simulink model "SIM"  (R2020b)
settings: Solver=ode1  StartTime=0.0  StopTime=inf  FixedStep=0.005  RelTol=1e-3
values from neighbouring files (symbols this model uses):
  previous_input_to_hidden_layer = rand (K,1)* 0.2 - 0.1    [preparation.m]
  TableSIN = [0 0.0549778488291 0.109955562006 0.164933003878 0.219910038795 0.274886531105 0.32986234516 0.384837345313 0.439811395917 0.494784361331 0.549756105914 0.604726494028 ... (5001 elements, 5001x1)]    [TableSIN.mat]
  weights_Qj_model = rand (S,K)* 0.2 - 0.1    [preparation.m]
  weights_W2 = rand ( K+1 , R ) * 0.2 - 0.1    [preparation.m]
  weights_W3 = rand ( R+1 , W ) * 0.2 - 0.1    [preparation.m]
  weights_Wd_model = rand (K,1)* 0.2 - 0.1    [preparation.m]
  weights_Y1_model = rand (K,1)* 0.2 - 0.1    [preparation.m]
  weigths_W1 = rand ( S+1 , K ) * 0.2 - 0.1    [preparation.m]
undefined symbols (not defined in the file or in its folder): D, I, N, P, scaling_a, scaling_b, SkalB, SkalG, strengthening_PID, weights_W1_Model, weights_W2_Model, weights_Xj, WzmocnienieDoWyjscia
libraries: bur_blks x111, pid_lib x3
(part 1 of 2)
settings Model: SimulationMode=external  Creator=barte  LastModifiedBy=barte
settings DataIOCC: SaveFormat=Array  SaveOutput=off  SignalLogging=off  DSMLogging=off  SaveTime=off  ReturnWorkspaceOutputs=off
settings OptimizationCC: OptimizeBlockIOStorage=off  EnableMemcpy=off  InitFltsAndDblsToZero=on  LifeSpan=inf
settings DebuggingCC: UnderspecifiedInitializationDetection=Classic  MergeDetectMultiDrivingBlocksExec=none  SolverPrmCheckMsg=warning  InheritedTsInSrcMsg=none  FcnCallInpInsideContextMsg=warning  FrameProcessingCompatibilityMsg=none  ModelReferenceSymbolNameMessage=none  StateNameClashWarn=warning  SFUnexpectedBacktrackingDiag=warning  SFNoUnconditionalDefaultTransitionDiag=warning
settings HardwareCC: ProdBitPerPointer=32  ProdBitPerSizeT=32  ProdBitPerPtrDiffT=32  ProdLargestAtomicFloat=None  ProdWordSize=32  ProdHWDeviceType=Intel->x86/Pentium
settings ModelReferenceCC: UpdateModelReferenceTargets=IfOutOfDate  ModelReferencePassRootInputsByReference=off  PropagateSignalLabelsOutOfModel=off
settings RTWCC: Description=B&R Automation Studio Target (GRT based)  SystemTargetFile=bur_grt.tlc  GenerateMakefile=off  TemplateMakefile=bur.tmf  RTWVerbose=off  TargetLang=C++
settings STFCustomTargetCC: TargetLangStandard=C++03 (ISO)  ParMdlRefBuildCompliant=on  ConcurrentExecutionCompliant=off  CPPClassGenCompliant=off  SystemTargetFile=bur_grt.tlc
settings GRTTargetCC: TargetLangStandard=C++03 (ISO)  CompOptLevelCompliant=off  ConcurrentExecutionCompliant=off  CombineOutputUpdateFcns=off  MatFileLogging=off  CPPClassGenCompliant=off  GRTInterface=on  UseToolchainInfoCompliant=off  ExtMode=on  ExtModeStaticAlloc=on  ExtModeStaticAllocSize=100000000  ExtModeMexArgs='192.168.0.10' 0 11159

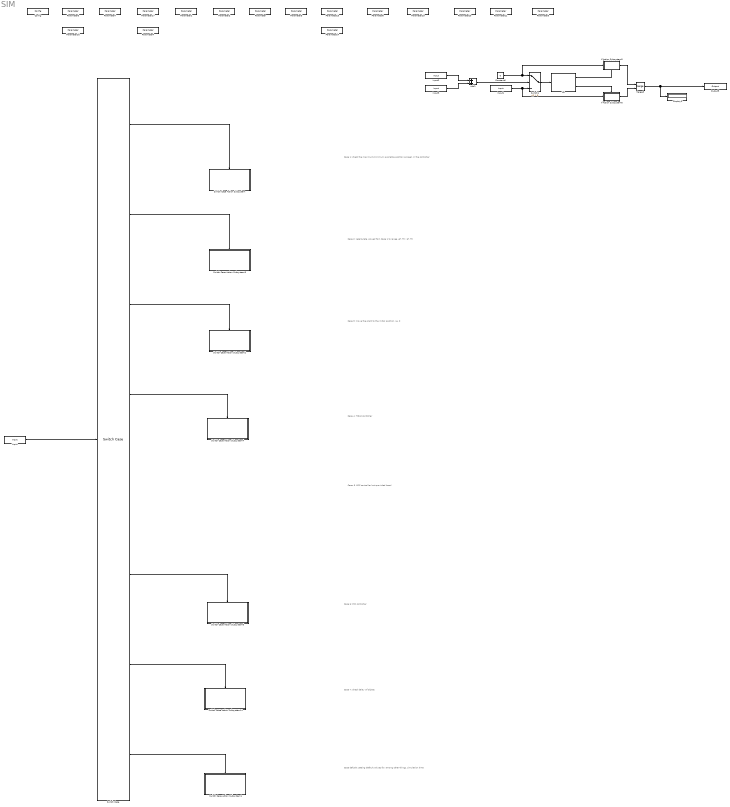
== system SIM ==
  note: Case: 5 MPC controller (not provided here)
  note: Case 4: HDLC controller
  note: Case 6: PID controller
  note: Case 7: check delay of object
  note: Case defualt: setting default values for, among other things, simulation time
  note: Case 1: check the maximum/minimum available position as seen in the controller
  note: Case 2: recalculate values from Case 1 to range -67.75 : 67.75
  note: Case 3: move the plant to the initial position i.e. 0
  Add1 : Sum
  Config : bur_blks/Config  Tag=Coder: GRT C++ Target: Task  bur_configset_ert=C - Code Generation (Embedded Real Time Target based)  bur_configset_grt=C - Code Generation (Generic Real Time Target based)  bur_maskHandle=-1
      settings: AttributesFormatString=%<Tag>  SourceProductName=B&R Automation Studio Toolbox
  Constant6 : Constant  Value=0
  Display3 : Display
  If Action Subsystem5 : Subsystem  TreatAsAtomicUnit=on
  If Action Subsystem6 : Subsystem  TreatAsAtomicUnit=on
  If3 : If  IfExpression=u1 == 0
  Input : bur_blks/Input  Tag=LOCAL LREAL Case  bur_var_name=Case  bur_scope=LOCAL  bur_data_type=LREAL  bur_init_value=0  bur_init_value_bool=FALSE  bur_array_index=0  bur_var_memory=standard  bur_in_parameter=off  bur_array_index_string=0
      settings: AttributesFormatString=%<Tag>  SourceProductName=B&R Automation Studio Toolbox
  Input1 : bur_blks/Input  Tag=LOCAL LREAL Case  bur_var_name=Case  bur_scope=LOCAL  bur_data_type=LREAL  bur_init_value=0  bur_init_value_bool=FALSE  bur_array_index=0  bur_var_memory=standard  bur_in_parameter=off  bur_array_index_string=0
      settings: AttributesFormatString=%<Tag>  SourceProductName=B&R Automation Studio Toolbox
  Input2 : bur_blks/Input  Tag=LOCAL LREAL STOP  bur_var_name=STOP  bur_scope=LOCAL  bur_data_type=LREAL  bur_init_value=0  bur_init_value_bool=FALSE  bur_array_index=0  bur_var_memory=standard  bur_in_parameter=off  bur_array_index_string=0
      settings: AttributesFormatString=%<Tag>  SourceProductName=B&R Automation Studio Toolbox
  Input3 : bur_blks/Input  Tag=LOCAL LREAL STOP_W  bur_var_name=STOP_W  bur_scope=LOCAL  bur_data_type=LREAL  bur_init_value=0  bur_init_value_bool=FALSE  bur_array_index=0  bur_var_memory=standard  bur_in_parameter=off  bur_array_index_string=0
      settings: AttributesFormatString=%<Tag>  SourceProductName=B&R Automation Studio Toolbox
  Merge3 : Merge
  Output5 : bur_blks/Output  Tag=LOCAL LREAL Case  bur_var_name=Case  bur_scope=LOCAL  bur_data_type=LREAL  bur_init_value=0  bur_init_value_bool=FALSE  bur_array_index=0  bur_var_memory=standard  bur_array_index_string=0
      settings: AttributesFormatString=%<Tag>  SourceProductName=B&R Automation Studio Toolbox
  Parameter : bur_blks/Parameter  Tag=LOCAL LREAL time  Priority=2147483646  bur_var_name=time  bur_scope=LOCAL  bur_data_type=LREAL  bur_init_value=-0.001  bur_init_value_bool=FALSE  bur_array_index=0  bur_old_var_name=T_symulacji  bur_var_memory=standard  bur_AS_string=time : LREAL := -0.001; (**)  bur_array_index_string=0
      settings: AttributesFormatString=%<Tag>  SourceProductName=B&R Automation Studio Toolbox
  Parameter1 : bur_blks/Parameter  Tag=LOCAL LREAL max_output  Priority=2147483646  bur_var_name=max_output  bur_scope=LOCAL  bur_data_type=LREAL  bur_init_value=0  bur_init_value_bool=FALSE  bur_array_index=0  bur_old_var_name=MAXOutput  bur_var_memory=standard  bur_AS_string=max_output : LREAL := 0; (**)  bur_array_index_string=0
      settings: AttributesFormatString=%<Tag>  SourceProductName=B&R Automation Studio Toolbox
  Parameter16 : bur_blks/Parameter  Tag=LOCAL INT a_output  Priority=2147483646  bur_var_name=a_output  bur_scope=LOCAL  bur_data_type=INT  bur_init_value=0  bur_init_value_bool=FALSE  bur_array_index=0  bur_old_var_name=AOutput  bur_var_memory=standard  bur_AS_string=a_output : INT := 0; (**)  bur_array_index_string=0
      settings: AttributesFormatString=%<Tag>  SourceProductName=B&R Automation Studio Toolbox
  Parameter17 : bur_blks/Parameter  Tag=LOCAL DINT strengthening_PID  Priority=2147483646  bur_var_name=strengthening_PID  bur_scope=LOCAL  bur_data_type=DINT  bur_init_value=32767  bur_init_value_bool=FALSE  bur_array_index=0  bur_old_var_name=strengthening_  bur_var_memory=standard  bur_array_index_string=1
      settings: AttributesFormatString=%<Tag>  SourceProductName=B&R Automation Studio Toolbox
  Parameter19 : bur_blks/Parameter  Tag=LOCAL LREAL I  Priority=2147483646  bur_var_name=I  bur_scope=LOCAL  bur_data_type=LREAL  bur_init_value=31.35  bur_init_value_bool=FALSE  bur_array_index=0  bur_old_var_name=P1  bur_var_memory=standard  bur_array_index_string=0
      settings: AttributesFormatString=%<Tag>  SourceProductName=B&R Automation Studio Toolbox
  Parameter2 : bur_blks/Parameter  Tag=LOCAL LREAL min_output  Priority=2147483646  bur_var_name=min_output  bur_scope=LOCAL  bur_data_type=LREAL  bur_init_value=0  bur_init_value_bool=FALSE  bur_array_index=0  bur_old_var_name=MINOutput  bur_var_memory=standard  bur_AS_string=min_output : LREAL := 0; (**)  bur_array_index_string=0
      settings: AttributesFormatString=%<Tag>  SourceProductName=B&R Automation Studio Toolbox
  Parameter20 : bur_blks/Parameter  Tag=LOCAL LREAL D  Priority=2147483646  bur_var_name=D  bur_scope=LOCAL  bur_data_type=LREAL  bur_init_value=0.00828  bur_init_value_bool=FALSE  bur_array_index=0  bur_old_var_name=I1  bur_var_memory=standard  bur_array_index_string=0
      settings: AttributesFormatString=%<Tag>  SourceProductName=B&R Automation Studio Toolbox
  Parameter21 : bur_blks/Parameter  Tag=LOCAL LREAL N  Priority=2147483646  bur_var_name=N  bur_scope=LOCAL  bur_data_type=LREAL  bur_init_value=1  bur_init_value_bool=FALSE  bur_array_index=0  bur_old_var_name=D1  bur_var_memory=standard  bur_array_index_string=0
      settings: AttributesFormatString=%<Tag>  SourceProductName=B&R Automation Studio Toolbox
  Parameter23 : bur_blks/Parameter  Tag=LOCAL LREAL scaling_a  Priority=2147483646  bur_var_name=scaling_a  bur_scope=LOCAL  bur_data_type=LREAL  bur_init_value=0  bur_init_value_bool=FALSE  bur_array_index=0  bur_old_var_name=SkalG  bur_var_memory=standard  bur_AS_string=scaling_a : LREAL := 0; (**)  bur_array_index_string=0
      settings: AttributesFormatString=%<Tag>  SourceProductName=B&R Automation Studio Toolbox
  Parameter24 : bur_blks/Parameter  Tag=LOCAL LREAL scaling_b  Priority=2147483646  bur_var_name=scaling_b  bur_scope=LOCAL  bur_data_type=LREAL  bur_init_value=0  bur_init_value_bool=FALSE  bur_array_index=0  bur_old_var_name=SkalB  bur_var_memory=standard  bur_AS_string=scaling_b : LREAL := 0; (**)  bur_array_index_string=0
      settings: AttributesFormatString=%<Tag>  SourceProductName=B&R Automation Studio Toolbox
  Parameter3 : bur_blks/Parameter  Tag=LOCAL LREAL step  Priority=2147483646  bur_var_name=step  bur_scope=LOCAL  bur_data_type=LREAL  bur_init_value=0.002  bur_init_value_bool=FALSE  bur_array_index=0  bur_old_var_name=Step  bur_var_memory=standard  bur_AS_string=step : LREAL := 0.002; (**)  bur_array_index_string=0
      settings: AttributesFormatString=%<Tag>  SourceProductName=B&R Automation Studio Toolbox
  Parameter4 : bur_blks/Parameter  Tag=LOCAL LREAL Case2  Priority=2147483646  bur_var_name=Case2  bur_scope=LOCAL  bur_data_type=LREAL  bur_init_value=0  bur_init_value_bool=FALSE  bur_array_index=0  bur_old_var_name=Parameter1  bur_var_memory=standard  bur_array_index_string=0
      settings: AttributesFormatString=%<Tag>  SourceProductName=B&R Automation Studio Toolbox
  Parameter5 : bur_blks/Parameter  Tag=LOCAL LREAL object_delay  Priority=2147483646  bur_var_name=object_delay  bur_scope=LOCAL  bur_data_type=LREAL  bur_init_value=4  bur_init_value_bool=FALSE  bur_array_index=0  bur_var_memory=standard  bur_AS_string=object_delay : LREAL := 4; (**)  bur_array_index_string=0
      settings: AttributesFormatString=%<Tag>  SourceProductName=B&R Automation Studio Toolbox
  Parameter6 : bur_blks/Parameter  Tag=LOCAL INT a_input  Priority=2147483646  bur_var_name=a_input  bur_scope=LOCAL  bur_data_type=INT  bur_init_value=0  bur_init_value_bool=FALSE  bur_array_index=0  bur_old_var_name=AInput  bur_var_memory=standard  bur_AS_string=a_input : INT := 0; (**)  bur_array_index_string=0
      settings: AttributesFormatString=%<Tag>  SourceProductName=B&R Automation Studio Toolbox
  Parameter7 : bur_blks/Parameter  Tag=LOCAL LREAL normalisation  Priority=2147483646  bur_var_name=normalisation  bur_scope=LOCAL  bur_data_type=LREAL  bur_init_value=70  bur_init_value_bool=FALSE  bur_array_index=0  bur_old_var_name=Normalisation  bur_var_memory=standard  bur_AS_string=normalisation : LREAL := 70; (**)  bur_array_index_string=0
      settings: AttributesFormatString=%<Tag>  SourceProductName=B&R Automation Studio Toolbox
  Parameter8 : bur_blks/Parameter  Tag=LOCAL LREAL P  Priority=2147483646  bur_var_name=P  bur_scope=LOCAL  bur_data_type=LREAL  bur_init_value=130.00  bur_init_value_bool=FALSE  bur_array_index=0  bur_old_var_name=I1  bur_var_memory=standard  bur_array_index_string=0
      settings: AttributesFormatString=%<Tag>  SourceProductName=B&R Automation Studio Toolbox
  Switch Case : SwitchCase  CaseConditions={1,2,3,4,5,6,7}
  Switch Case Action Subsystem : Subsystem  TreatAsAtomicUnit=on
  Switch Case Action Subsystem1 : Subsystem  TreatAsAtomicUnit=on
  Switch Case Action Subsystem14 : Subsystem  TreatAsAtomicUnit=on
  Switch Case Action Subsystem2 : Subsystem  TreatAsAtomicUnit=on
  Switch Case Action Subsystem3 : Subsystem  TreatAsAtomicUnit=on
  Switch Case Action Subsystem4 : Subsystem  TreatAsAtomicUnit=on
  Switch Case Action Subsystem6 : Subsystem  TreatAsAtomicUnit=on
  Switch1 : Switch  Criteria=u2 > Threshold
  wires:
  Input/1 -> Switch Case/1
  Switch Case/1 -> Switch Case Action Subsystem/Action
  If Action Subsystem6/1(Out1) -> Merge3/2
  If3/1 -> If Action Subsystem5/Action
  Input3/1 -> Add1/2
  Input2/1 -> Add1/1
  If3/2 -> If Action Subsystem6/Action
  Switch1/1 -> If3/1
  Add1/1 -> Switch1/2
  Input1/1 -> If Action Subsystem6/1(In1), Switch1/3
  Constant6/1 -> If Action Subsystem5/1(In1), Switch1/1
  If Action Subsystem5/1(Out1) -> Merge3/1
  Merge3/1 -> Display3/1, Output5/1
  Switch Case/8 -> Switch Case Action Subsystem1/Action
  Switch Case/3 -> Switch Case Action Subsystem2/Action
  Switch Case/2 -> Switch Case Action Subsystem3/Action
  Switch Case/4 -> Switch Case Action Subsystem4/Action
  Switch Case/6 -> Switch Case Action Subsystem6/Action
  Switch Case/7 -> Switch Case Action Subsystem14/Action

== system SIM/If Action Subsystem5 ==
  In1 : Inport
  Action Port : ActionPort  ActionPortLabel=if(u1 == 0)
  Out1 : Outport
  wires:
  In1/1 -> Out1/1

== system SIM/If Action Subsystem6 ==
  In1 : Inport
  Action Port : ActionPort  ActionPortLabel=else
  Out1 : Outport
  wires:
  In1/1 -> Out1/1

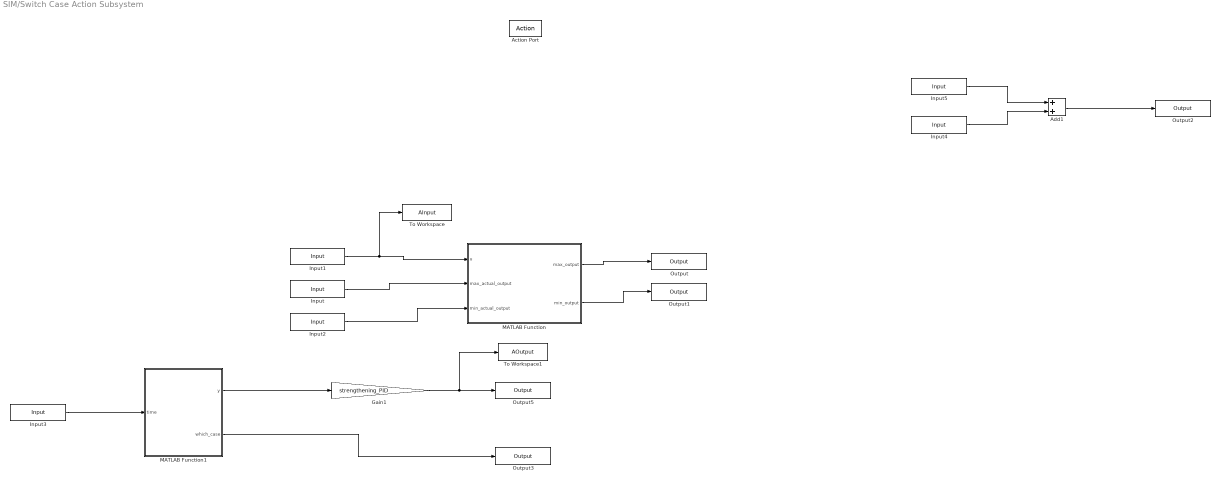
== system SIM/Switch Case Action Subsystem ==
  Action Port : ActionPort  ActionPortLabel=case [ 1 ]:
  Add1 : Sum
  Gain1 : Gain  Gain=strengthening_PID
  Input : bur_blks/Input  Tag=LOCAL LREAL max_output  bur_var_name=max_output  bur_scope=LOCAL  bur_data_type=LREAL  bur_init_value=0  bur_init_value_bool=FALSE  bur_array_index=0  bur_var_memory=standard  bur_in_parameter=off  bur_AS_string=max_output : LREAL := 0; (**)  bur_array_index_string=0
      settings: AttributesFormatString=%<Tag>  SourceProductName=B&R Automation Studio Toolbox
  Input1 : bur_blks/Input  Tag=LOCAL LREAL a_input  bur_var_name=a_input  bur_scope=LOCAL  bur_data_type=LREAL  bur_init_value=0  bur_init_value_bool=FALSE  bur_array_index=0  bur_var_memory=standard  bur_in_parameter=off  bur_AS_string=a_input : LREAL := 0; (**)  bur_array_index_string=0
      settings: AttributesFormatString=%<Tag>  SourceProductName=B&R Automation Studio Toolbox
  Input2 : bur_blks/Input  Tag=LOCAL LREAL max_output  bur_var_name=max_output  bur_scope=LOCAL  bur_data_type=LREAL  bur_init_value=0  bur_init_value_bool=FALSE  bur_array_index=0  bur_var_memory=standard  bur_in_parameter=off  bur_AS_string=max_output : LREAL := 0; (**)  bur_array_index_string=0
      settings: AttributesFormatString=%<Tag>  SourceProductName=B&R Automation Studio Toolbox
  Input3 : bur_blks/Input  Tag=LOCAL LREAL time  bur_var_name=time  bur_scope=LOCAL  bur_data_type=LREAL  bur_init_value=0  bur_init_value_bool=FALSE  bur_array_index=0  bur_var_memory=standard  bur_in_parameter=off  bur_AS_string=time : LREAL := 0; (**)  bur_array_index_string=0
      settings: AttributesFormatString=%<Tag>  SourceProductName=B&R Automation Studio Toolbox
  Input4 : bur_blks/Input  Tag=LOCAL LREAL time  bur_var_name=time  bur_scope=LOCAL  bur_data_type=LREAL  bur_init_value=0  bur_init_value_bool=FALSE  bur_array_index=0  bur_var_memory=standard  bur_in_parameter=off  bur_AS_string=time : LREAL := 0; (**)  bur_array_index_string=0
      settings: AttributesFormatString=%<Tag>  SourceProductName=B&R Automation Studio Toolbox
  Input5 : bur_blks/Input  Tag=LOCAL REAL step  bur_var_name=step  bur_scope=LOCAL  bur_data_type=REAL  bur_init_value=0  bur_init_value_bool=FALSE  bur_array_index=0  bur_var_memory=standard  bur_in_parameter=off  bur_AS_string=step : REAL := 0; (**)  bur_array_index_string=0
      settings: AttributesFormatString=%<Tag>  SourceProductName=B&R Automation Studio Toolbox
  MATLAB Function : MATLAB Function  TreatAsAtomicUnit=on
  MATLAB Function1 : MATLAB Function  TreatAsAtomicUnit=on
  Output : bur_blks/Output  Tag=LOCAL LREAL max_output  bur_var_name=max_output  bur_scope=LOCAL  bur_data_type=LREAL  bur_init_value=0  bur_init_value_bool=FALSE  bur_array_index=0  bur_var_memory=standard  bur_AS_string=max_output : LREAL := 0; (**)  bur_array_index_string=0
      settings: AttributesFormatString=%<Tag>  SourceProductName=B&R Automation Studio Toolbox
  Output1 : bur_blks/Output  Tag=LOCAL LREAL min_output  bur_var_name=min_output  bur_scope=LOCAL  bur_data_type=LREAL  bur_init_value=0  bur_init_value_bool=FALSE  bur_array_index=0  bur_var_memory=standard  bur_AS_string=min_output : LREAL := 0; (**)  bur_array_index_string=0
      settings: AttributesFormatString=%<Tag>  SourceProductName=B&R Automation Studio Toolbox
  Output2 : bur_blks/Output  Tag=LOCAL LREAL time  bur_var_name=time  bur_scope=LOCAL  bur_data_type=LREAL  bur_init_value=0  bur_init_value_bool=FALSE  bur_array_index=0  bur_var_memory=standard  bur_AS_string=time : LREAL := 0; (**)  bur_array_index_string=0
      settings: AttributesFormatString=%<Tag>  SourceProductName=B&R Automation Studio Toolbox
  Output3 : bur_blks/Output  Tag=LOCAL LREAL Case  bur_var_name=Case  bur_scope=LOCAL  bur_data_type=LREAL  bur_init_value=0  bur_init_value_bool=FALSE  bur_array_index=0  bur_var_memory=standard  bur_array_index_string=0
      settings: AttributesFormatString=%<Tag>  SourceProductName=B&R Automation Studio Toolbox
  Output5 : bur_blks/Output  Tag=LOCAL LREAL a_output  bur_var_name=a_output  bur_scope=LOCAL  bur_data_type=LREAL  bur_init_value=0  bur_init_value_bool=FALSE  bur_array_index=0  bur_var_memory=standard  bur_AS_string=a_output : LREAL := 0; (**)  bur_array_index_string=0
      settings: AttributesFormatString=%<Tag>  SourceProductName=B&R Automation Studio Toolbox
  To Workspace : ToWorkspace  VariableName=AInput  SampleTime=-1
  To Workspace1 : ToWorkspace  VariableName=AOutput  SampleTime=-1
  wires:
  Gain1/1 -> To Workspace1/1, Output5/1
  Input1/1 -> To Workspace/1, MATLAB Function/1(u)
  Input/1 -> MATLAB Function/2(max_actual_output)
  MATLAB Function/1(max_output) -> Output/1
  MATLAB Function/2(min_output) -> Output1/1
  Input2/1 -> MATLAB Function/3(min_actual_output)
  Input4/1 -> Add1/2
  Input5/1 -> Add1/1
  Add1/1 -> Output2/1
  Input3/1 -> MATLAB Function1/1(time)
  MATLAB Function1/1(y) -> Gain1/1
  MATLAB Function1/2(which_case) -> Output3/1

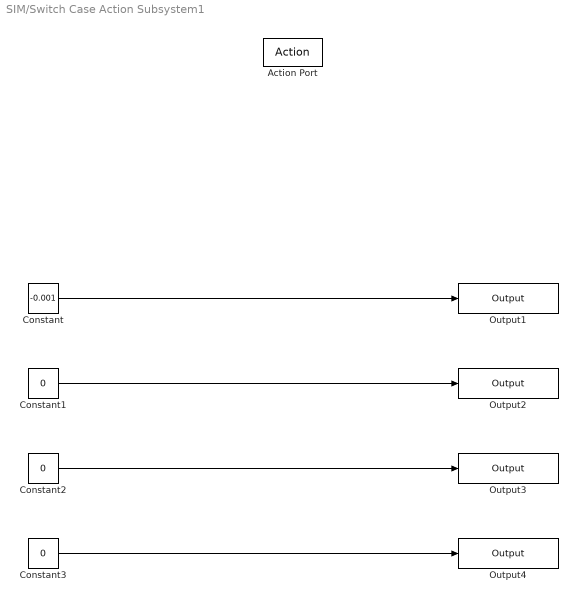
== system SIM/Switch Case Action Subsystem1 ==
  Action Port : ActionPort  ActionPortLabel=default:
  Constant : Constant  Value=-0.001
  Constant1 : Constant  Value=0
  Constant2 : Constant  Value=0
  Constant3 : Constant  Value=0
  Output1 : bur_blks/Output  Tag=LOCAL LREAL time  bur_var_name=time  bur_scope=LOCAL  bur_data_type=LREAL  bur_init_value=0  bur_init_value_bool=FALSE  bur_array_index=0  bur_var_memory=standard  bur_AS_string=time : LREAL := 0; (**)  bur_array_index_string=0
      settings: AttributesFormatString=%<Tag>  SourceProductName=B&R Automation Studio Toolbox
  Output2 : bur_blks/Output  Tag=LOCAL LREAL STOP  bur_var_name=STOP  bur_scope=LOCAL  bur_data_type=LREAL  bur_init_value=0  bur_init_value_bool=FALSE  bur_array_index=0  bur_var_memory=standard  bur_array_index_string=0
      settings: AttributesFormatString=%<Tag>  SourceProductName=B&R Automation Studio Toolbox
  Output3 : bur_blks/Output  Tag=LOCAL LREAL STOP_W  bur_var_name=STOP_W  bur_scope=LOCAL  bur_data_type=LREAL  bur_init_value=0  bur_init_value_bool=FALSE  bur_array_index=0  bur_var_memory=standard  bur_array_index_string=0
      settings: AttributesFormatString=%<Tag>  SourceProductName=B&R Automation Studio Toolbox
  Output4 : bur_blks/Output  Tag=LOCAL LREAL Case2  bur_var_name=Case2  bur_scope=LOCAL  bur_data_type=LREAL  bur_init_value=0  bur_init_value_bool=FALSE  bur_array_index=0  bur_var_memory=standard  bur_array_index_string=0
      settings: AttributesFormatString=%<Tag>  SourceProductName=B&R Automation Studio Toolbox
  wires:
  Constant/1 -> Output1/1
  Constant1/1 -> Output2/1
  Constant2/1 -> Output3/1
  Constant3/1 -> Output4/1

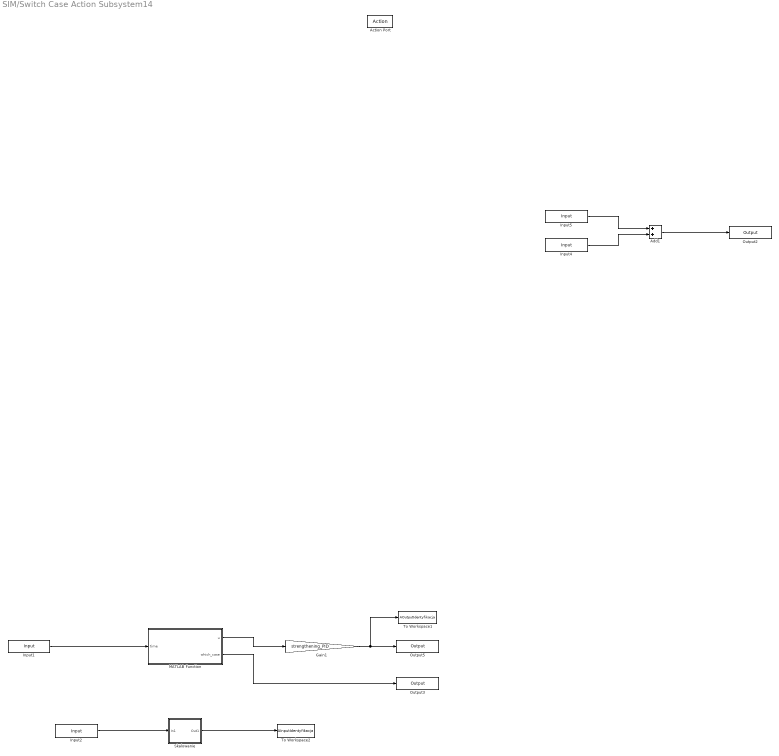
== system SIM/Switch Case Action Subsystem14 ==
  Action Port : ActionPort  ActionPortLabel=case [ 7 ]:
  Add1 : Sum
  Gain1 : Gain  Gain=strengthening_PID
  Input1 : bur_blks/Input  Tag=LOCAL LREAL time  bur_var_name=time  bur_scope=LOCAL  bur_data_type=LREAL  bur_init_value=0  bur_init_value_bool=FALSE  bur_array_index=0  bur_var_memory=standard  bur_in_parameter=off  bur_AS_string=time : LREAL := 0; (**)  bur_array_index_string=0
      settings: AttributesFormatString=%<Tag>  SourceProductName=B&R Automation Studio Toolbox
  Input2 : bur_blks/Input  Tag=LOCAL LREAL a_input  bur_var_name=a_input  bur_scope=LOCAL  bur_data_type=LREAL  bur_init_value=0  bur_init_value_bool=FALSE  bur_array_index=0  bur_var_memory=standard  bur_in_parameter=off  bur_AS_string=a_input : LREAL := 0; (**)  bur_array_index_string=0
      settings: AttributesFormatString=%<Tag>  SourceProductName=B&R Automation Studio Toolbox
  Input4 : bur_blks/Input  Tag=LOCAL LREAL T_symulacji  bur_var_name=T_symulacji  bur_scope=LOCAL  bur_data_type=LREAL  bur_init_value=0  bur_init_value_bool=FALSE  bur_array_index=0  bur_var_memory=standard  bur_in_parameter=off  bur_array_index_string=0
      settings: AttributesFormatString=%<Tag>  SourceProductName=B&R Automation Studio Toolbox
  Input5 : bur_blks/Input  Tag=LOCAL REAL Krok  bur_var_name=Krok  bur_scope=LOCAL  bur_data_type=REAL  bur_init_value=0  bur_init_value_bool=FALSE  bur_array_index=0  bur_var_memory=standard  bur_in_parameter=off  bur_array_index_string=0
      settings: AttributesFormatString=%<Tag>  SourceProductName=B&R Automation Studio Toolbox
  MATLAB Function : MATLAB Function  TreatAsAtomicUnit=on
  Output2 : bur_blks/Output  Tag=LOCAL LREAL T_symulacji  bur_var_name=T_symulacji  bur_scope=LOCAL  bur_data_type=LREAL  bur_init_value=0  bur_init_value_bool=FALSE  bur_array_index=0  bur_var_memory=standard  bur_array_index_string=0
      settings: AttributesFormatString=%<Tag>  SourceProductName=B&R Automation Studio Toolbox
  Output3 : bur_blks/Output  Tag=LOCAL LREAL Case  bur_var_name=Case  bur_scope=LOCAL  bur_data_type=LREAL  bur_init_value=0  bur_init_value_bool=FALSE  bur_array_index=0  bur_var_memory=standard  bur_array_index_string=0
      settings: AttributesFormatString=%<Tag>  SourceProductName=B&R Automation Studio Toolbox
  Output5 : bur_blks/Output  Tag=LOCAL LREAL a_output  bur_var_name=a_output  bur_scope=LOCAL  bur_data_type=LREAL  bur_init_value=0  bur_init_value_bool=FALSE  bur_array_index=0  bur_var_memory=standard  bur_AS_string=a_output : LREAL := 0; (**)  bur_array_index_string=0
      settings: AttributesFormatString=%<Tag>  SourceProductName=B&R Automation Studio Toolbox
  Skalowanie : Subsystem
  To Workspace1 : ToWorkspace  VariableName=AOutputIdentyfikacja  SampleTime=-1
  To Workspace2 : ToWorkspace  VariableName=AInputIdentyfikacja  SampleTime=-1
  wires:
  Input5/1 -> Add1/1
  Input4/1 -> Add1/2
  Add1/1 -> Output2/1
  Input1/1 -> MATLAB Function/1(time)
  Gain1/1 -> To Workspace1/1, Output5/1
  MATLAB Function/1(u) -> Gain1/1
  MATLAB Function/2(which_case) -> Output3/1
  Input2/1 -> Skalowanie/1(In1)
  Skalowanie/1(Out1) -> To Workspace2/1

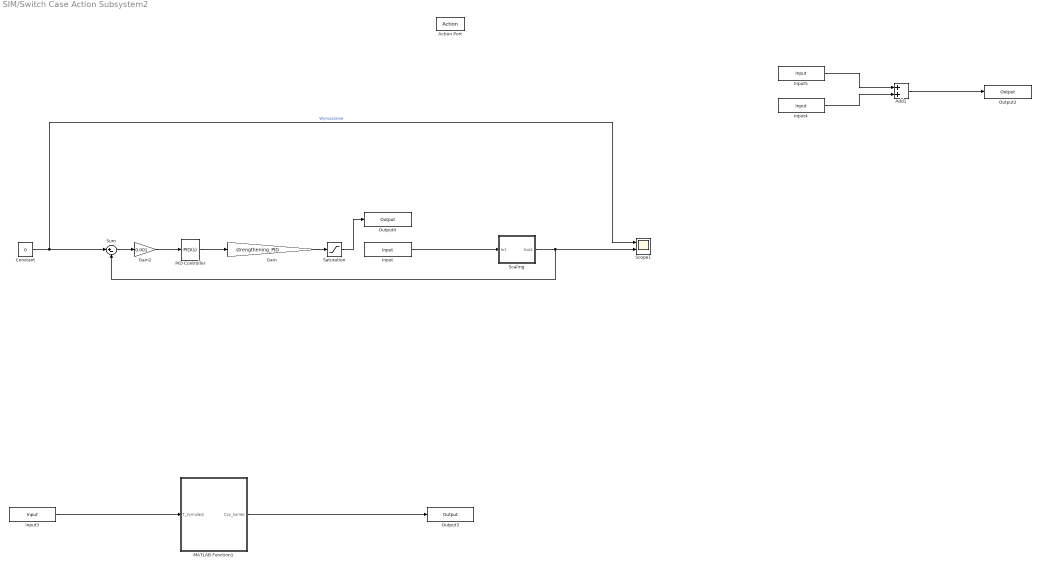
== system SIM/Switch Case Action Subsystem2 ==
  Action Port : ActionPort  ActionPortLabel=case [ 3 ]:
  Add1 : Sum
  Constant : Constant  Value=0
  Gain : Gain  Gain=strengthening_PID
  Gain2 : Gain  Gain=0.001
  Input : bur_blks/Input  Tag=LOCAL LREAL a_input  bur_var_name=a_input  bur_scope=LOCAL  bur_data_type=LREAL  bur_init_value=0  bur_init_value_bool=FALSE  bur_array_index=0  bur_var_memory=standard  bur_in_parameter=off  bur_AS_string=a_input : LREAL := 0; (**)  bur_array_index_string=0
      settings: AttributesFormatString=%<Tag>  SourceProductName=B&R Automation Studio Toolbox
  Input3 : bur_blks/Input  Tag=LOCAL LREAL time  bur_var_name=time  bur_scope=LOCAL  bur_data_type=LREAL  bur_init_value=0  bur_init_value_bool=FALSE  bur_array_index=0  bur_var_memory=standard  bur_in_parameter=off  bur_AS_string=time : LREAL := 0; (**)  bur_array_index_string=0
      settings: AttributesFormatString=%<Tag>  SourceProductName=B&R Automation Studio Toolbox
  Input4 : bur_blks/Input  Tag=LOCAL LREAL time  bur_var_name=time  bur_scope=LOCAL  bur_data_type=LREAL  bur_init_value=0  bur_init_value_bool=FALSE  bur_array_index=0  bur_var_memory=standard  bur_in_parameter=off  bur_AS_string=time : LREAL := 0; (**)  bur_array_index_string=0
      settings: AttributesFormatString=%<Tag>  SourceProductName=B&R Automation Studio Toolbox
  Input5 : bur_blks/Input  Tag=LOCAL REAL step  bur_var_name=step  bur_scope=LOCAL  bur_data_type=REAL  bur_init_value=0  bur_init_value_bool=FALSE  bur_array_index=0  bur_var_memory=standard  bur_in_parameter=off  bur_AS_string=step : REAL := 0; (**)  bur_array_index_string=0
      settings: AttributesFormatString=%<Tag>  SourceProductName=B&R Automation Studio Toolbox
  MATLAB Function1 : MATLAB Function  TreatAsAtomicUnit=on
  Output2 : bur_blks/Output  Tag=LOCAL LREAL time  bur_var_name=time  bur_scope=LOCAL  bur_data_type=LREAL  bur_init_value=0  bur_init_value_bool=FALSE  bur_array_index=0  bur_var_memory=standard  bur_AS_string=time : LREAL := 0; (**)  bur_array_index_string=0
      settings: AttributesFormatString=%<Tag>  SourceProductName=B&R Automation Studio Toolbox
  Output3 : bur_blks/Output  Tag=LOCAL LREAL STOP  bur_var_name=STOP  bur_scope=LOCAL  bur_data_type=LREAL  bur_init_value=0  bur_init_value_bool=FALSE  bur_array_index=0  bur_var_memory=standard  bur_array_index_string=0
      settings: AttributesFormatString=%<Tag>  SourceProductName=B&R Automation Studio Toolbox
  Output4 : bur_blks/Output  Tag=LOCAL LREAL a_output  bur_var_name=a_output  bur_scope=LOCAL  bur_data_type=LREAL  bur_init_value=0  bur_init_value_bool=FALSE  bur_array_index=0  bur_var_memory=standard  bur_AS_string=a_output : LREAL := 0; (**)  bur_array_index_string=0
      settings: AttributesFormatString=%<Tag>  SourceProductName=B&R Automation Studio Toolbox
  PID Controller : pid_lib/PID Controller  Controller=PID  Form=Parallel  TimeDomain=Continuous-time  UseExternalTs=off  SampleTime=-1  IntegratorMethod=Forward Euler  FilterMethod=Forward Euler  ControllerParametersSource=internal  P=P  I=I  D=D  UseFilter=on  N=N  TunerSelectOption=Transfer Function Based (PID Tuner App)  InitialConditionSource=internal  InitialConditionForIntegrator=0  InitialConditionForFilter=0  DifferentiatorICPrevScaledInput=0  ExternalReset=none  TrackingMode=off  Kt=1  LimitOutput=on  SatLimitsSource=internal  UpperSaturationLimit=1  LowerSaturationLimit=-1  LinearizeAsGain=on  AntiWindupMode=clamping  Kb=1  POutMin=[]  POutMax=[]  IOutMin=[]  IOutMax=[]  DOutMin=[]  DOutMax=[]  NOutMin=[]  NOutMax=[]  SumOutMin=[]  SumOutMax=[]  SaturationOutMin=[]  SaturationOutMax=[]  PParamMin=[]  PParamMax=[]  IParamMin=[]  IParamMax=[]  DParamMin=[]  DParamMax=[]  NParamMin=[]  NParamMax=[]  KbParamMin=[]  KbParamMax=[]  KtParamMin=[]  KtParamMax=[]  KbOutMin=[]  KbOutMax=[]  KtOutMin=[]  KtOutMax=[]  IntegratorOutMin=[]  IntegratorOutMax=[]  FilterOutMin=[]  FilterOutMax=[]  SumI1OutMin=[]  SumI1OutMax=[]  SumI2OutMin=[]  SumI2OutMax=[]  SumI3OutMin=[]  SumI3OutMax=[]  SumI4OutMin=[]  SumI4OutMax=[]  SumDOutMin=[]  SumDOutMax=[]  DifferentiatorOutMin=[]  DifferentiatorOutMax=[]  FilterDiffOutCoefMin=[]  FilterDiffOutCoefMax=[]  ReciprocalOutMin=[]  ReciprocalOutMax=[]  SumDenOutMin=[]  SumDenOutMax=[]  SumNumOutMin=[]  SumNumOutMax=[]  DivideOutMin=[]  DivideOutMax=[]  UdiffTsProdOutMin=[]  UdiffTsProdOutMax=[]  NTsProdOutMin=[]  NTsProdOutMax=[]  UintegralTsProdOutMin=[]  UintegralTsProdOutMax=[]  UngainTsProdOutMin=[]  UngainTsProdOutMax=[]  IntegratorContinuousStateAttributes=''  IntegratorStateMustResolveToSignalObject=off  IntegratorRTWStateStorageClass=Auto  FilterContinuousStateAttributes=''  FilterStateMustResolveToSignalObject=off  FilterRTWStateStorageClass=Auto  ParallelPVariant=InternalParameters  IdealPVariant=Disabled  IVariant=InternalParameters  DVariant=InternalParameters  IntegratorVariant=Continuous  SatVariant=Enabled  AWVariant=ContClampingParallel  PCopyVariant=Disabled  TRVariant=Disabled  FdbkBlocksVariant=Forward  IdealPFdbkVariant=Disabled  SatFdbkVariant=Disabled  DerivativeFilterVariant=ContFilter  NVariant=InternalParameters  NCopyVariant=Disabled  FilterICVariant=InternalICsFilter  IntegratorICVariant=InternalICs  ExternalResetVariant=Disabled  TRSumVariant=Passthrough  SumFdbkVariant=Disabled  SumVariant=Sum_PID  TsampFilterVariant=InternalTs  TsampNgainVariant=Passthrough  TsampIntegralVariant=Passthrough  ExternalSaturationOutDataTypeStr=Inherit: Same as second input
  Saturation : Saturate  UpperLimit=32767  LowerLimit=-32767
  Scaling : Subsystem
  Scope1 : Scope  NumInputPorts=2
  Sum : Sum  Inputs=|+-
  wires:
  Input4/1 -> Add1/2
  Input5/1 -> Add1/1
  Add1/1 -> Output2/1
  Input3/1 -> MATLAB Function1/1(T_symulacji)
  MATLAB Function1/1(Czy_koniec) -> Output3/1
  Saturation/1 -> Output4/1
  Sum/1 -> Gain2/1
  Gain2/1 -> PID Controller/1
  PID Controller/1 -> Gain/1
  Constant/1 -> Sum/1, Scope1/1  "Wymuszenie"
  Gain/1 -> Saturation/1
  Scaling/1(Out1) -> Sum/2, Scope1/2
  Input/1 -> Scaling/1(In1)

== system SIM/Switch Case Action Subsystem3 ==
  Action Port : ActionPort  ActionPortLabel=case [ 2 ]:
  Input : bur_blks/Input  Tag=LOCAL LREAL max_output  bur_var_name=max_output  bur_scope=LOCAL  bur_data_type=LREAL  bur_init_value=0  bur_init_value_bool=FALSE  bur_array_index=0  bur_var_memory=standard  bur_in_parameter=off  bur_AS_string=max_output : LREAL := 0; (**)  bur_array_index_string=0
      settings: AttributesFormatString=%<Tag>  SourceProductName=B&R Automation Studio Toolbox
  Input2 : bur_blks/Input  Tag=LOCAL LREAL min_output  bur_var_name=min_output  bur_scope=LOCAL  bur_data_type=LREAL  bur_init_value=0  bur_init_value_bool=FALSE  bur_array_index=0  bur_var_memory=standard  bur_in_parameter=off  bur_AS_string=min_output : LREAL := 0; (**)  bur_array_index_string=0
      settings: AttributesFormatString=%<Tag>  SourceProductName=B&R Automation Studio Toolbox
  MATLAB Function : MATLAB Function  TreatAsAtomicUnit=on
  Output1 : bur_blks/Output  Tag=LOCAL LREAL Case  bur_var_name=Case  bur_scope=LOCAL  bur_data_type=LREAL  bur_init_value=0  bur_init_value_bool=FALSE  bur_array_index=0  bur_var_memory=standard  bur_array_index_string=0
      settings: AttributesFormatString=%<Tag>  SourceProductName=B&R Automation Studio Toolbox
  Output3 : bur_blks/Output  Tag=LOCAL LREAL scaling_a  bur_var_name=scaling_a  bur_scope=LOCAL  bur_data_type=LREAL  bur_init_value=0  bur_init_value_bool=FALSE  bur_array_index=0  bur_var_memory=standard  bur_AS_string=scaling_a : LREAL := 0; (**)  bur_array_index_string=0
      settings: AttributesFormatString=%<Tag>  SourceProductName=B&R Automation Studio Toolbox
  Output6 : bur_blks/Output  Tag=LOCAL LREAL scaling_b  bur_var_name=scaling_b  bur_scope=LOCAL  bur_data_type=LREAL  bur_init_value=0  bur_init_value_bool=FALSE  bur_array_index=0  bur_var_memory=standard  bur_AS_string=scaling_b : LREAL := 0; (**)  bur_array_index_string=0
      settings: AttributesFormatString=%<Tag>  SourceProductName=B&R Automation Studio Toolbox
  wires:
  Input/1 -> MATLAB Function/1(max_output)
  MATLAB Function/1(scaling_a) -> Output3/1
  MATLAB Function/2(scaling_b) -> Output6/1
  Input2/1 -> MATLAB Function/2(min_output)
  MATLAB Function/3(which_case) -> Output1/1

== system SIM/Switch Case Action Subsystem4 ==
  Action Port : ActionPort  ActionPortLabel=case [ 4 ]:
  Input : bur_blks/Input  Tag=LOCAL LREAL Case2  bur_var_name=Case2  bur_scope=LOCAL  bur_data_type=LREAL  bur_init_value=0  bur_init_value_bool=FALSE  bur_array_index=0  bur_var_memory=standard  bur_in_parameter=off  bur_array_index_string=0
      settings: AttributesFormatString=%<Tag>  SourceProductName=B&R Automation Studio Toolbox
  Switch Case : SwitchCase  CaseConditions={1,2}
  Switch Case Action Subsystem1 : Subsystem  TreatAsAtomicUnit=on
  Switch Case Action Subsystem3 : Subsystem  TreatAsAtomicUnit=on
  Switch Case Action Subsystem4 : Subsystem  TreatAsAtomicUnit=on
  wires:
  Input/1 -> Switch Case/1
  Switch Case/1 -> Switch Case Action Subsystem4/Action
  Switch Case/2 -> Switch Case Action Subsystem1/Action
  Switch Case/3 -> Switch Case Action Subsystem3/Action

== system SIM/Switch Case Action Subsystem6 ==
  Action Port : ActionPort  ActionPortLabel=case [ 6 ]:
  Input : bur_blks/Input  Tag=LOCAL LREAL Case2  bur_var_name=Case2  bur_scope=LOCAL  bur_data_type=LREAL  bur_init_value=0  bur_init_value_bool=FALSE  bur_array_index=0  bur_var_memory=standard  bur_in_parameter=off  bur_array_index_string=0
      settings: AttributesFormatString=%<Tag>  SourceProductName=B&R Automation Studio Toolbox
  Switch Case : SwitchCase  CaseConditions={1,2,3}
  Switch Case Action Subsystem1 : Subsystem  TreatAsAtomicUnit=on
  Switch Case Action Subsystem2 : Subsystem  TreatAsAtomicUnit=on
  Switch Case Action Subsystem3 : Subsystem  TreatAsAtomicUnit=on
  Switch Case Action Subsystem4 : Subsystem  TreatAsAtomicUnit=on
  wires:
  Input/1 -> Switch Case/1
  Switch Case/1 -> Switch Case Action Subsystem4/Action
  Switch Case/2 -> Switch Case Action Subsystem1/Action
  Switch Case/4 -> Switch Case Action Subsystem3/Action
  Switch Case/3 -> Switch Case Action Subsystem2/Action

== system SIM/Switch Case Action Subsystem14/Skalowanie ==
  In1 : Inport
  Add : Sum
  Constant : Constant  Value=SkalB
  Gain : Gain  Gain=SkalG
  Out1 : Outport
  wires:
  In1/1 -> Gain/1
  Gain/1 -> Add/2
  Add/1 -> Out1/1
  Constant/1 -> Add/1

== system SIM/Switch Case Action Subsystem2/Scaling ==
  In1 : Inport
  Add : Sum
  Constant : Constant  Value=scaling_b
  Gain : Gain  Gain=scaling_a
  Out1 : Outport
  wires:
  In1/1 -> Gain/1
  Gain/1 -> Add/2
  Add/1 -> Out1/1
  Constant/1 -> Add/1

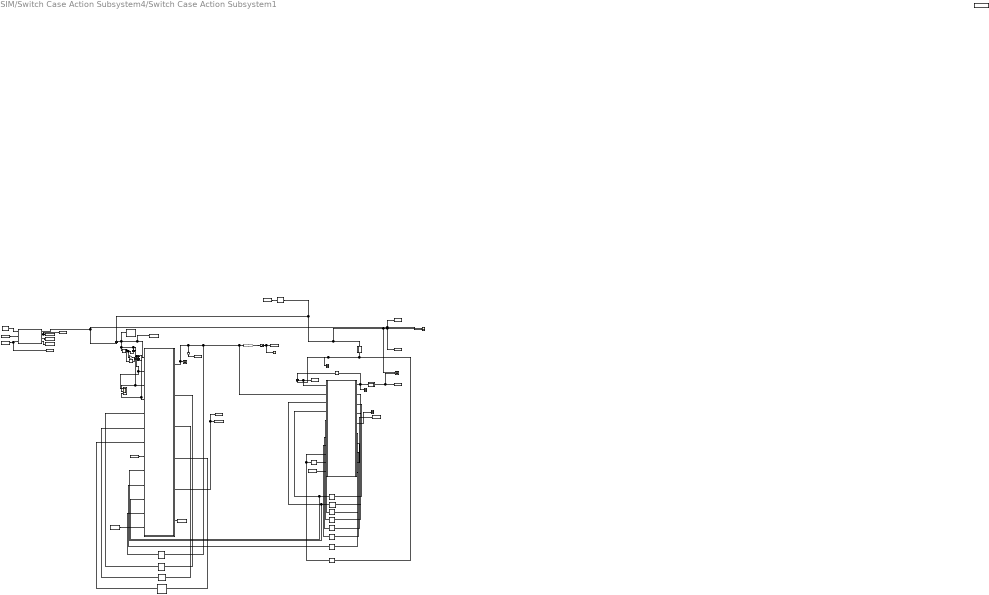
== system SIM/Switch Case Action Subsystem4/Switch Case Action Subsystem1 ==
  Action Port : ActionPort  ActionPortLabel=case [ 2 ]:
  Add5 : Sum  Inputs=+-+
  Constant12 : Constant  Value=TableSIN
  Constant14 : Constant  Value=75000
  DRNN : MATLAB Function  TreatAsAtomicUnit=on
  Delay{59,61..62,65} (4 alike) : Delay  DelayLength=1
  Delay60 : Delay  DelayLength=1  InitialCondition=weights_W3
  Delay63 : Delay  DelayLength=1  InitialCondition=weights_W2_Model
  Delay64 : Delay  DelayLength=1  InitialCondition=weights_W1_Model
  Delay69 : Delay  DelayLength=1  InitialCondition=weights_Y1_model
  Delay70 : Delay  DelayLength=1  InitialCondition=weights_Xj
  Delay71 : Delay  DelayLength=1  InitialCondition=weights_Wd_model
  Delay72 : Delay  DelayLength=1  InitialCondition=previous_input_to_hidden_layer
  Delay73 : Delay  DelayLength=1  InitialCondition=weights_Qj_model
  Delay74 : Delay  DelayLength=1  InitialCondition=0.5
  Delay75 : Delay  DelayLength=1  InitialCondition=weigths_W1
  Delay76 : Delay  DelayLength=1  InitialCondition=weights_W2
  Delay77 : Delay  DelayLength=1  InitialCondition=0
  Denormalisation : Subsystem
  Gain11 : Gain  Gain=WzmocnienieDoWyjscia
  Gain13 : Gain  Gain=10
  Gain14 : Gain  Gain=2
  Indicators of regulatory quality : Subsystem
  Input22 : bur_blks/Input  Tag=LOCAL REAL time_iterator  bur_var_name=time_iterator  bur_scope=LOCAL  bur_data_type=REAL  bur_init_value=-0.001  bur_init_value_bool=FALSE  bur_array_index=0  bur_var_memory=standard  bur_in_parameter=off  bur_AS_string=time_iterator : REAL := -0.001; (**)  bur_array_index_string=0
      settings: AttributesFormatString=%<Tag>  SourceProductName=B&R Automation Studio Toolbox
  Input23 : bur_blks/Input  Tag=LOCAL LREAL table_iterator  bur_var_name=table_iterator  bur_scope=LOCAL  bur_data_type=LREAL  bur_init_value=0  bur_init_value_bool=FALSE  bur_array_index=0  bur_var_memory=standard  bur_in_parameter=off  bur_AS_string=table_iterator : LREAL := 0; (**)  bur_array_index_string=0
      settings: AttributesFormatString=%<Tag>  SourceProductName=B&R Automation Studio Toolbox
  Input24 : bur_blks/Input  Tag=LOCAL LREAL IteracjaHDLNNC2  bur_var_name=IteracjaHDLNNC2  bur_scope=LOCAL  bur_data_type=LREAL  bur_init_value=1  bur_init_value_bool=FALSE  bur_array_index=0  bur_var_memory=standard  bur_in_parameter=off  bur_array_index_string=0
      settings: AttributesFormatString=%<Tag>  SourceProductName=B&R Automation Studio Toolbox
  Input25 : bur_blks/Input  Tag=LOCAL LREAL DRNN_iteration  bur_var_name=DRNN_iteration  bur_scope=LOCAL  bur_data_type=LREAL  bur_init_value=1  bur_init_value_bool=FALSE  bur_array_index=0  bur_var_memory=standard  bur_in_parameter=off  bur_AS_string=DRNN_iteration : LREAL := 1; (**)  bur_array_index_string=0
      settings: AttributesFormatString=%<Tag>  SourceProductName=B&R Automation Studio Toolbox
  Input26 : bur_blks/Input  Tag=LOCAL LREAL a_input  bur_var_name=a_input  bur_scope=LOCAL  bur_data_type=LREAL  bur_init_value=0  bur_init_value_bool=FALSE  bur_array_index=0  bur_var_memory=standard  bur_in_parameter=off  bur_AS_string=a_input : LREAL := 0; (**)  bur_array_index_string=0
      settings: AttributesFormatString=%<Tag>  SourceProductName=B&R Automation Studio Toolbox
  NARX - Lypunov learning rate old bias HDLNNC - 3 layers7 : MATLAB Function  TreatAsAtomicUnit=on
  Normalisation : Subsystem
  Output30 : bur_blks/Output  Tag=LOCAL REAL time_iterator  bur_var_name=time_iterator  bur_scope=LOCAL  bur_data_type=REAL  bur_init_value=0  bur_init_value_bool=FALSE  bur_array_index=0  bur_var_memory=standard  bur_AS_string=time_iterator : REAL := 0; (**)  bur_array_index_string=0
      settings: AttributesFormatString=%<Tag>  SourceProductName=B&R Automation Studio Toolbox
  Output31 : bur_blks/Output  Tag=LOCAL LREAL table_iterator  bur_var_name=table_iterator  bur_scope=LOCAL  bur_data_type=LREAL  bur_init_value=0  bur_init_value_bool=FALSE  bur_array_index=0  bur_var_memory=standard  bur_AS_string=table_iterator : LREAL := 0; (**)  bur_array_index_string=0
      settings: AttributesFormatString=%<Tag>  SourceProductName=B&R Automation Studio Toolbox
  Output32 : bur_blks/Output  Tag=LOCAL LREAL Case  bur_var_name=Case  bur_scope=LOCAL  bur_data_type=LREAL  bur_init_value=0  bur_init_value_bool=FALSE  bur_array_index=0  bur_var_memory=standard  bur_AS_string=Case : LREAL := 0; (**)  bur_array_index_string=0
      settings: AttributesFormatString=%<Tag>  SourceProductName=B&R Automation Studio Toolbox
  Output33 : bur_blks/Output  Tag=LOCAL LREAL HDLC_iteration  bur_var_name=HDLC_iteration  bur_scope=LOCAL  bur_data_type=LREAL  bur_init_value=0  bur_init_value_bool=FALSE  bur_array_index=0  bur_var_memory=standard  bur_AS_string=HDLC_iteration : LREAL := 0; (**)  bur_array_index_string=0
      settings: AttributesFormatString=%<Tag>  SourceProductName=B&R Automation Studio Toolbox
  Output34 : bur_blks/Output  Tag=LOCAL LREAL DRNN_iteration  bur_var_name=DRNN_iteration  bur_scope=LOCAL  bur_data_type=LREAL  bur_init_value=1  bur_init_value_bool=FALSE  bur_array_index=0  bur_var_memory=standard  bur_AS_string=DRNN_iteration : LREAL := 1; (**)  bur_array_index_string=0
      settings: AttributesFormatString=%<Tag>  SourceProductName=B&R Automation Studio Toolbox
  Output35 : bur_blks/Output  Tag=LOCAL LREAL HDLC_mse  bur_var_name=HDLC_mse  bur_scope=LOCAL  bur_data_type=LREAL  bur_init_value=0  bur_init_value_bool=FALSE  bur_array_index=0  bur_var_memory=standard  bur_AS_string=HDLC_mse : LREAL := 0; (**)  bur_array_index_string=0
      settings: AttributesFormatString=%<Tag>  SourceProductName=B&R Automation Studio Toolbox
  Output36 : bur_blks/Output  Tag=LOCAL LREAL a_output  bur_var_name=a_output  bur_scope=LOCAL  bur_data_type=LREAL  bur_init_value=0  bur_init_value_bool=FALSE  bur_array_index=0  bur_var_memory=standard  bur_AS_string=a_output : LREAL := 0; (**)  bur_array_index_string=0
      settings: AttributesFormatString=%<Tag>  SourceProductName=B&R Automation Studio Toolbox
  Saturation4 : Saturate  UpperLimit=32767  LowerLimit=-32767
  Scope{26,28,31,33..34} (5 alike) : Scope
  Scope27 : Scope  NumInputPorts=2
  Scope29 : Scope  NumInputPorts=2
  Scope32 : Scope  NumInputPorts=3
  Skalowanie3 : Subsystem
  Sum10 : Sum  Inputs=-+
  Sum11 : Sum  Inputs=-+
  Sum12 : Sum  Inputs=+-
  To Workspace35 : ToWorkspace  VariableName=SPHDLNNC  SampleTime=-1
  To Workspace36 : ToWorkspace  VariableName=PVmodelHDLNNC  SampleTime=-1
  To Workspace37 : ToWorkspace  VariableName=control_error  SampleTime=-1
  To Workspace38 : ToWorkspace  VariableName=ErrorModelu  SampleTime=-1
  To Workspace39 : ToWorkspace  VariableName=PVobiektuHDLNNC  SampleTime=-1
  To Workspace40 : ToWorkspace  VariableName=MSEHDLNNC  SampleTime=-1
      settings: MaxDataPoints=1
  To Workspace41 : ToWorkspace  VariableName=Iterator  SampleTime=-1
  To Workspace42 : ToWorkspace  VariableName=IteratorCzasu  SampleTime=-1
  To Workspace43 : ToWorkspace  VariableName=u  SampleTime=-1
  Wyjscie5 : MATLAB Function  TreatAsAtomicUnit=on
  wires:
  Delay75/1 -> NARX - Lypunov learning rate old bias HDLNNC - 3 layers7/5(old_weights_W1_HDL)
  Constant12/1 -> Wyjscie5/1(TableSIN)
  NARX - Lypunov learning rate old bias HDLNNC - 3 layers7/5(MSEOUT) -> To Workspace40/1, Output35/1
  Wyjscie5/3(iteration_out_table) -> Output31/1
  Normalisation/1(Out1) -> Scope34/1, Sum11/2, Delay74/1
  Wyjscie5/4(which_case) -> Output32/1
  Gain14/1 -> Add5/2
  DRNN/8(Qj_after) -> Delay73/1
  Delay60/1 -> NARX - Lypunov learning rate old bias HDLNNC - 3 layers7/7(old_weights_W3_HDL)
  Input26/1 -> Skalowanie3/1(In1)
  Gain11/1 -> Saturation4/1
  Input24/1 -> NARX - Lypunov learning rate old bias HDLNNC - 3 layers7/8(iteration_before)
  Delay64/1 -> DRNN/3(weights_W1), NARX - Lypunov learning rate old bias HDLNNC - 3 layers7/9(weights_of_DRNN_W1)
  Wyjscie5/1(output_value) -> Sum10/2, To Workspace35/1, Scope29/2  "Obiekt"
  DRNN/6(Xj_after) -> Delay70/1
  Gain13/1 -> To Workspace43/1
  NARX - Lypunov learning rate old bias HDLNNC - 3 layers7/6(iteration_after_calculation) -> Output33/1
  Sum10/1 -> Indicators of regulatory quality/1(Error), Delay61/1, NARX - Lypunov learning rate old bias HDLNNC - 3 layers7/2(ud1), Scope32/1, Add5/1, Sum12/1, To Workspace37/1, NARX - Lypunov learning rate old bias HDLNNC - 3 layers7/1(E)
  Delay61/1 -> Delay62/1, Gain14/1, Sum12/2
  Delay63/1 -> DRNN/4(weights_W2), NARX - Lypunov learning rate old bias HDLNNC - 3 layers7/11(weights_of_DRNN_W2)
  Delay77/1 -> NARX - Lypunov learning rate old bias HDLNNC - 3 layers7/12(previous_output)
  Sum11/1 -> To Workspace38/1, DRNN/1(E)
  NARX - Lypunov learning rate old bias HDLNNC - 3 layers7/1(u) -> Gain13/1, Gain11/1, DRNN/2(reference_signal), Delay77/1, Scope28/1  "u"
  DRNN/7(Pj_after) -> Delay72/1
  NARX - Lypunov learning rate old bias HDLNNC - 3 layers7/4(new_weights_W3_HDL) -> Delay60/1
  Constant14/1 -> NARX - Lypunov learning rate old bias HDLNNC - 3 layers7/13(total_iteration)
  Add5/1 -> NARX - Lypunov learning rate old bias HDLNNC - 3 layers7/4(ud3), Scope32/3
  Delay65/1 -> DRNN/10(previous_output_of_object_d2)
  Delay72/1 -> DRNN/7(previous_input_to_hidden_layer)
  Input23/1 -> To Workspace41/1, Wyjscie5/3(iteration_in_table)
  Wyjscie5/2(iteration_out) -> To Workspace42/1, Output30/1
  Delay76/1 -> NARX - Lypunov learning rate old bias HDLNNC - 3 layers7/6(old_weights_W2_HDL)
  NARX - Lypunov learning rate old bias HDLNNC - 3 layers7/2(new_weights_W1_HDL) -> Delay75/1
  Input25/1 -> DRNN/11(iteration_before)
  Delay73/1 -> DRNN/8(weights_Qj_model)
  DRNN/3(weights_W2_after) -> Delay63/1
  DRNN/5(MSEOUT) -> Scope31/1
  DRNN/1(y) -> Delay59/1, Denormalisation/1(u), Scope33/1  "PV model"
  DRNN/9(iteration_after) -> Output34/1
  Delay62/1 -> Add5/3
  Sum12/1 -> NARX - Lypunov learning rate old bias HDLNNC - 3 layers7/3(ud2), Scope32/2
  DRNN/2(weights_W1_after) -> Delay64/1
  Delay74/1 -> DRNN/9(previous_output_of_object_d1), Delay65/1
  Delay69/1 -> NARX - Lypunov learning rate old bias HDLNNC - 3 layers7/10(output_of_model)
  Input22/1 -> Wyjscie5/2(iteration_in)
  Delay71/1 -> DRNN/5(weights_Wd_model)
  DRNN/10(output_of_hidden_layer) -> Delay69/1
  Saturation4/1 -> Scope26/1, Output36/1
  Delay70/1 -> DRNN/6(weights_Xj_model)
  Delay59/1 -> Sum11/1
  DRNN/4(weights_Wd_after) -> Delay71/1
  Skalowanie3/1(Out1) -> Scope27/1, To Workspace39/1, Scope29/1, Normalisation/1(In1), Sum10/1  "PV"
  NARX - Lypunov learning rate old bias HDLNNC - 3 layers7/3(new_weights_W2_HDL) -> Delay76/1
  Denormalisation/1(Xods) -> Scope27/2, To Workspace36/1

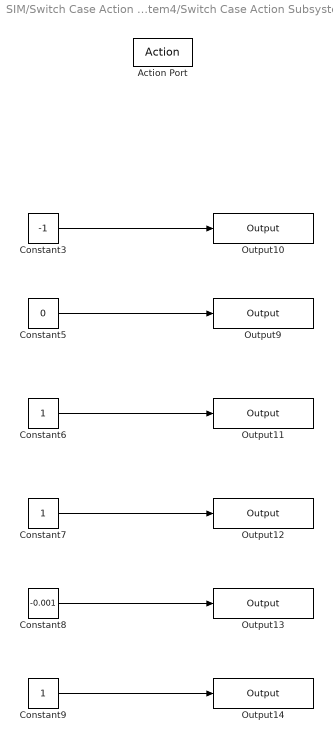
== system SIM/Switch Case Action Subsystem4/Switch Case Action Subsystem3 ==
  Action Port : ActionPort  ActionPortLabel=default:
  Constant3 : Constant  Value=-1
  Constant5 : Constant  Value=0
  Constant6 : Constant
  Constant7 : Constant
  Constant8 : Constant  Value=-0.001
  Constant9 : Constant
  Output10 : bur_blks/Output  Tag=LOCAL LREAL time_iterator  bur_var_name=time_iterator  bur_scope=LOCAL  bur_data_type=LREAL  bur_init_value=0  bur_init_value_bool=FALSE  bur_array_index=0  bur_var_memory=standard  bur_AS_string=time_iterator : LREAL := 0; (**)  bur_array_index_string=0
      settings: AttributesFormatString=%<Tag>  SourceProductName=B&R Automation Studio Toolbox
  Output11 : bur_blks/Output  Tag=LOCAL LREAL HDLC_iteration  bur_var_name=HDLC_iteration  bur_scope=LOCAL  bur_data_type=LREAL  bur_init_value=0  bur_init_value_bool=FALSE  bur_array_index=0  bur_var_memory=standard  bur_AS_string=HDLC_iteration : LREAL := 0; (**)  bur_array_index_string=0
      settings: AttributesFormatString=%<Tag>  SourceProductName=B&R Automation Studio Toolbox
  Output12 : bur_blks/Output  Tag=LOCAL LREAL DRNN_iteration  bur_var_name=DRNN_iteration  bur_scope=LOCAL  bur_data_type=LREAL  bur_init_value=1  bur_init_value_bool=FALSE  bur_array_index=0  bur_var_memory=standard  bur_AS_string=DRNN_iteration : LREAL := 1; (**)  bur_array_index_string=0
      settings: AttributesFormatString=%<Tag>  SourceProductName=B&R Automation Studio Toolbox
  Output13 : bur_blks/Output  Tag=LOCAL LREAL time  bur_var_name=time  bur_scope=LOCAL  bur_data_type=LREAL  bur_init_value=0  bur_init_value_bool=FALSE  bur_array_index=0  bur_var_memory=standard  bur_AS_string=time : LREAL := 0; (**)  bur_array_index_string=0
      settings: AttributesFormatString=%<Tag>  SourceProductName=B&R Automation Studio Toolbox
  Output14 : bur_blks/Output  Tag=LOCAL LREAL table_sq_iterator  bur_var_name=table_sq_iterator  bur_scope=LOCAL  bur_data_type=LREAL  bur_init_value=0  bur_init_value_bool=FALSE  bur_array_index=0  bur_var_memory=standard  bur_AS_string=table_sq_iterator : LREAL := 0; (**)  bur_array_index_string=0
      settings: AttributesFormatString=%<Tag>  SourceProductName=B&R Automation Studio Toolbox
  Output9 : bur_blks/Output  Tag=LOCAL LREAL table_iterator  bur_var_name=table_iterator  bur_scope=LOCAL  bur_data_type=LREAL  bur_init_value=0  bur_init_value_bool=FALSE  bur_array_index=0  bur_var_memory=standard  bur_AS_string=table_iterator : LREAL := 0; (**)  bur_array_index_string=0
      settings: AttributesFormatString=%<Tag>  SourceProductName=B&R Automation Studio Toolbox
  wires:
  Constant3/1 -> Output10/1
  Constant5/1 -> Output9/1
  Constant6/1 -> Output11/1
  Constant7/1 -> Output12/1
  Constant8/1 -> Output13/1
  Constant9/1 -> Output14/1

== system SIM/Switch Case Action Subsystem4/Switch Case Action Subsystem4 ==
  Action Port : ActionPort  ActionPortLabel=case [ 1 ]:
  Constant : Constant  Value=0
  Output : bur_blks/Output  Tag=LOCAL LREAL Case2  bur_var_name=Case2  bur_scope=LOCAL  bur_data_type=LREAL  bur_init_value=0  bur_init_value_bool=FALSE  bur_array_index=0  bur_var_memory=standard  bur_array_index_string=0
      settings: AttributesFormatString=%<Tag>  SourceProductName=B&R Automation Studio Toolbox
  wires:
  Constant/1 -> Output/1
